simulink model "Microgrid_transition_model_111821_ben"  (R2020a)
settings: Solver=VariableStepAuto  StartTime=0.0  StopTime=20  MaxStep=1e-4  RelTol=1e-3
PreLoadFcn:
  | %run('FC_microgrid_param.m')
  | %load('gen_grid_init.mat')
InitFcn:
  | %load myisoModel_init;
  | run('FC_microgrid_param.m')
  | tic
  | run('CARTinitFcn.m')
  | %caseNo = 2;
  | 
  | %if (caseNo == 1)
  | %set_param(['Isolated_grid_paper_model_022521/SignalGen'], 'ActiveScenario', 'PStep222kW');
  | %else
  | %set_param(['Isolated_grid_paper_model_022521/SignalGen'], 'ActiveScenario', 'QStep222kVAr');
  | 
  | %end;
StopFcn:
  | toc
undefined symbols (not defined in the file): breakpoints1, breakpoints2, cc_kp, cp_table_data, ctrl, D1, Delta, DiscIntNeverNeededParam, DT, FC_BESS, FC_PV_FirstSolar, find_system, gcbh, libFC_BESS, libFC_PV, LowerLimit, magnitude, oversize, pll_ki, pll_kp, pq_ts, sps_rtmsupport, timer, ts, Ts, Ts_APC, Ts_Control, Ts_Power, UpperLimit
libraries: powerlib x152, powerlib_extras x100, simulink x95, powerlib_meascontrol x86, eePowerMeasurement x26, pi_ctrl x16, simulink_extras x12, sps_avr x7, spsDieselMotorModel x3, libFSArray x2, SignalEditorBlockLib x2, libLgBattery x1
(part 4 of 14)

== system Microgrid_transition_model_111821_ben/Defferable Load (0-446.25 kW)/Resistive Loads ==
  Bit 0 : powerlib/Elements/Three-Phase Parallel RLC Load  LConnTagsString=A|B|C  Configuration=Y (grounded)  NominalVoltage=Vphase_phase_lissage  Vabc=[1e3 1e3 1e3]  Vabcp=[1e3 1e3 1e3]  NominalFrequency=Freq  UnbalancedPower=off  ActivePower=P_lissage_min  InductivePower=0  CapacitivePower=0  Pabc=[10e3 9e3 11e3]  QLabc=[100 90 110]  QCabc=[100 90 110]  Pabcp=[10e3 9e3 11e3]  QLabcp=[100 90 110]  QCabcp=[100 90 110]  Measurements=None  LoadType=constant Z
      settings: SourceProductBaseCode=MT,PS
  Bit 1 : powerlib/Elements/Three-Phase Parallel RLC Load  LConnTagsString=A|B|C  Configuration=Y (grounded)  NominalVoltage=Vphase_phase_lissage  Vabc=[1e3 1e3 1e3]  Vabcp=[1e3 1e3 1e3]  NominalFrequency=Freq  UnbalancedPower=off  ActivePower=2*P_lissage_min  InductivePower=0  CapacitivePower=0  Pabc=[10e3 9e3 11e3]  QLabc=[100 90 110]  QCabc=[100 90 110]  Pabcp=[10e3 9e3 11e3]  QLabcp=[100 90 110]  QCabcp=[100 90 110]  Measurements=None  LoadType=constant Z
      settings: SourceProductBaseCode=MT,PS
  Bit 2 : powerlib/Elements/Three-Phase Parallel RLC Load  LConnTagsString=A|B|C  Configuration=Y (grounded)  NominalVoltage=Vphase_phase_lissage  Vabc=[1e3 1e3 1e3]  Vabcp=[1e3 1e3 1e3]  NominalFrequency=Freq  UnbalancedPower=off  ActivePower=2^2*P_lissage_min  InductivePower=0  CapacitivePower=0  Pabc=[10e3 9e3 11e3]  QLabc=[100 90 110]  QCabc=[100 90 110]  Pabcp=[10e3 9e3 11e3]  QLabcp=[100 90 110]  QCabcp=[100 90 110]  Measurements=None  LoadType=constant Z
      settings: SourceProductBaseCode=MT,PS
  Bit 3 : powerlib/Elements/Three-Phase Parallel RLC Load  LConnTagsString=A|B|C  Configuration=Y (grounded)  NominalVoltage=Vphase_phase_lissage  Vabc=[1e3 1e3 1e3]  Vabcp=[1e3 1e3 1e3]  NominalFrequency=Freq  UnbalancedPower=off  ActivePower=2^3*P_lissage_min  InductivePower=0  CapacitivePower=0  Pabc=[10e3 9e3 11e3]  QLabc=[100 90 110]  QCabc=[100 90 110]  Pabcp=[10e3 9e3 11e3]  QLabcp=[100 90 110]  QCabcp=[100 90 110]  Measurements=None  LoadType=constant Z
      settings: SourceProductBaseCode=MT,PS
  Bit 4 : powerlib/Elements/Three-Phase Parallel RLC Load  LConnTagsString=A|B|C  Configuration=Y (grounded)  NominalVoltage=Vphase_phase_lissage  Vabc=[1e3 1e3 1e3]  Vabcp=[1e3 1e3 1e3]  NominalFrequency=Freq  UnbalancedPower=off  ActivePower=2^4*P_lissage_min  InductivePower=0  CapacitivePower=0  Pabc=[10e3 9e3 11e3]  QLabc=[100 90 110]  QCabc=[100 90 110]  Pabcp=[10e3 9e3 11e3]  QLabcp=[100 90 110]  QCabcp=[100 90 110]  Measurements=None  LoadType=constant Z
      settings: SourceProductBaseCode=MT,PS
  Bit 5 : powerlib/Elements/Three-Phase Parallel RLC Load  LConnTagsString=A|B|C  Configuration=Y (grounded)  NominalVoltage=Vphase_phase_lissage  Vabc=[1e3 1e3 1e3]  Vabcp=[1e3 1e3 1e3]  NominalFrequency=Freq  UnbalancedPower=off  ActivePower=2^5*P_lissage_min  InductivePower=0  CapacitivePower=0  Pabc=[10e3 9e3 11e3]  QLabc=[100 90 110]  QCabc=[100 90 110]  Pabcp=[10e3 9e3 11e3]  QLabcp=[100 90 110]  QCabcp=[100 90 110]  Measurements=None  LoadType=constant Z
      settings: SourceProductBaseCode=MT,PS
  Bit 6 : powerlib/Elements/Three-Phase Parallel RLC Load  LConnTagsString=A|B|C  Configuration=Y (grounded)  NominalVoltage=Vphase_phase_lissage  Vabc=[1e3 1e3 1e3]  Vabcp=[1e3 1e3 1e3]  NominalFrequency=Freq  UnbalancedPower=off  ActivePower=2^6*P_lissage_min  InductivePower=0  CapacitivePower=0  Pabc=[10e3 9e3 11e3]  QLabc=[100 90 110]  QCabc=[100 90 110]  Pabcp=[10e3 9e3 11e3]  QLabcp=[100 90 110]  QCabcp=[100 90 110]  Measurements=None  LoadType=constant Z
      settings: SourceProductBaseCode=MT,PS
  Bit 7 : powerlib/Elements/Three-Phase Parallel RLC Load  LConnTagsString=A|B|C  Configuration=Y (grounded)  NominalVoltage=Vphase_phase_lissage  Vabc=[1e3 1e3 1e3]  Vabcp=[1e3 1e3 1e3]  NominalFrequency=Freq  UnbalancedPower=off  ActivePower=2^7*P_lissage_min  InductivePower=0  CapacitivePower=0  Pabc=[10e3 9e3 11e3]  QLabc=[100 90 110]  QCabc=[100 90 110]  Pabcp=[10e3 9e3 11e3]  QLabcp=[100 90 110]  QCabcp=[100 90 110]  Measurements=None  LoadType=constant Z
      settings: SourceProductBaseCode=MT,PS
  A0 : PMIOPort  Side=Left
  B0 : PMIOPort  Port=2  Side=Left
  C0 : PMIOPort  Port=3  Side=Left
  A1 : PMIOPort  Port=4  Side=Left
  B1 : PMIOPort  Port=5  Side=Left
  C1 : PMIOPort  Port=6  Side=Left
  A2 : PMIOPort  Port=7  Side=Left
  B2 : PMIOPort  Port=8  Side=Left
  C2 : PMIOPort  Port=9  Side=Left
  A3 : PMIOPort  Port=10  Side=Left
  B3 : PMIOPort  Port=11  Side=Left
  C3 : PMIOPort  Port=12  Side=Left
  A4 : PMIOPort  Port=13  Side=Left
  B4 : PMIOPort  Port=14  Side=Left
  C4 : PMIOPort  Port=15  Side=Left
  A5 : PMIOPort  Port=16  Side=Left
  B5 : PMIOPort  Port=17  Side=Left
  C5 : PMIOPort  Port=18  Side=Left
  A6 : PMIOPort  Port=19  Side=Left
  B6 : PMIOPort  Port=20  Side=Left
  C6 : PMIOPort  Port=21  Side=Left
  A7 : PMIOPort  Port=22  Side=Left
  B7 : PMIOPort  Port=23  Side=Left
  C7 : PMIOPort  Port=24  Side=Left
  connections:
  C7/RConn1 -- Bit 7/LConn3
  B7/RConn1 -- Bit 7/LConn2
  A7/RConn1 -- Bit 7/LConn1
  C6/RConn1 -- Bit 6/LConn3
  B6/RConn1 -- Bit 6/LConn2
  A6/RConn1 -- Bit 6/LConn1
  C5/RConn1 -- Bit 5/LConn3
  B5/RConn1 -- Bit 5/LConn2
  A5/RConn1 -- Bit 5/LConn1
  C4/RConn1 -- Bit 4/LConn3
  B4/RConn1 -- Bit 4/LConn2
  A4/RConn1 -- Bit 4/LConn1
  C3/RConn1 -- Bit 3/LConn3
  B3/RConn1 -- Bit 3/LConn2
  A3/RConn1 -- Bit 3/LConn1
  C2/RConn1 -- Bit 2/LConn3
  B2/RConn1 -- Bit 2/LConn2
  A2/RConn1 -- Bit 2/LConn1
  C1/RConn1 -- Bit 1/LConn3
  B1/RConn1 -- Bit 1/LConn2
  A1/RConn1 -- Bit 1/LConn1
  C0/RConn1 -- Bit 0/LConn3
  B0/RConn1 -- Bit 0/LConn2
  A0/RConn1 -- Bit 0/LConn1

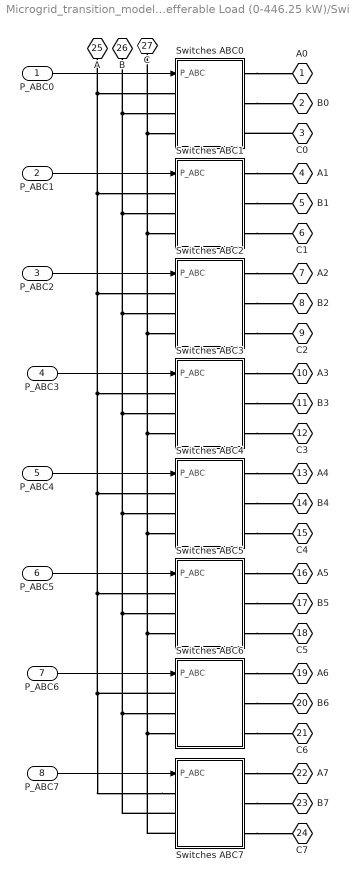
== system Microgrid_transition_model_111821_ben/Defferable Load (0-446.25 kW)/Switches ==
  P_ABC0 : Inport
  P_ABC1 : Inport  Port=2
  P_ABC2 : Inport  Port=3
  P_ABC3 : Inport  Port=4
  P_ABC4 : Inport  Port=5
  P_ABC5 : Inport  Port=6
  P_ABC6 : Inport  Port=7
  P_ABC7 : Inport  Port=8
  Switches ABC0 : Subsystem
  Switches ABC1 : Subsystem
  Switches ABC2 : Subsystem
  Switches ABC3 : Subsystem
  Switches ABC4 : Subsystem
  Switches ABC5 : Subsystem
  Switches ABC6 : Subsystem
  Switches ABC7 : Subsystem
  A0 : PMIOPort  Side=Right
  B0 : PMIOPort  Port=2  Side=Right
  C0 : PMIOPort  Port=3  Side=Right
  A1 : PMIOPort  Port=4  Side=Right
  B1 : PMIOPort  Port=5  Side=Right
  C1 : PMIOPort  Port=6  Side=Right
  A2 : PMIOPort  Port=7  Side=Right
  B2 : PMIOPort  Port=8  Side=Right
  C2 : PMIOPort  Port=9  Side=Right
  A3 : PMIOPort  Port=10  Side=Right
  B3 : PMIOPort  Port=11  Side=Right
  C3 : PMIOPort  Port=12  Side=Right
  A4 : PMIOPort  Port=13  Side=Right
  B4 : PMIOPort  Port=14  Side=Right
  C4 : PMIOPort  Port=15  Side=Right
  A5 : PMIOPort  Port=16  Side=Right
  B5 : PMIOPort  Port=17  Side=Right
  C5 : PMIOPort  Port=18  Side=Right
  A6 : PMIOPort  Port=19  Side=Right
  B6 : PMIOPort  Port=20  Side=Right
  C6 : PMIOPort  Port=21  Side=Right
  A7 : PMIOPort  Port=22  Side=Right
  B7 : PMIOPort  Port=23  Side=Right
  C7 : PMIOPort  Port=24  Side=Right
  A : PMIOPort  Port=25  Side=Left
  B : PMIOPort  Port=26  Side=Left
  C : PMIOPort  Port=27  Side=Left
  wires:
  P_ABC7/1 -> Switches ABC7/1(P_ABC)
  P_ABC6/1 -> Switches ABC6/1(P_ABC)
  P_ABC5/1 -> Switches ABC5/1(P_ABC)
  P_ABC4/1 -> Switches ABC4/1(P_ABC)
  P_ABC3/1 -> Switches ABC3/1(P_ABC)
  P_ABC2/1 -> Switches ABC2/1(P_ABC)
  P_ABC1/1 -> Switches ABC1/1(P_ABC)
  P_ABC0/1 -> Switches ABC0/1(P_ABC)
  connections:
  Switches ABC0/RConn1 -- A0/RConn1
  Switches ABC0/RConn2 -- B0/RConn1
  C0/RConn1 -- Switches ABC0/RConn3
  Switches ABC1/RConn1 -- A1/RConn1
  Switches ABC1/RConn2 -- B1/RConn1
  Switches ABC1/RConn3 -- C1/RConn1
  Switches ABC2/RConn1 -- A2/RConn1
  Switches ABC2/RConn2 -- B2/RConn1
  Switches ABC2/RConn3 -- C2/RConn1
  Switches ABC3/RConn1 -- A3/RConn1
  Switches ABC3/RConn2 -- B3/RConn1
  Switches ABC3/RConn3 -- C3/RConn1
  Switches ABC4/RConn1 -- A4/RConn1
  Switches ABC4/RConn2 -- B4/RConn1
  Switches ABC4/RConn3 -- C4/RConn1
  Switches ABC5/RConn1 -- A5/RConn1
  Switches ABC5/RConn2 -- B5/RConn1
  Switches ABC5/RConn3 -- C5/RConn1
  Switches ABC6/RConn1 -- A6/RConn1
  Switches ABC6/RConn2 -- B6/RConn1
  Switches ABC6/RConn3 -- C6/RConn1
  Switches ABC7/RConn3 -- C7/RConn1
  Switches ABC7/RConn2 -- B7/RConn1
  Switches ABC7/RConn1 -- A7/RConn1
  Switches ABC7/LConn2 -- Switches ABC0/LConn2 -- B/RConn1 -- Switches ABC1/LConn2 -- Switches ABC2/LConn2 -- Switches ABC3/LConn2 -- Switches ABC4/LConn2 -- Switches ABC5/LConn2 -- Switches ABC6/LConn2
  Switches ABC7/LConn3 -- Switches ABC0/LConn3 -- C/RConn1 -- Switches ABC1/LConn3 -- Switches ABC2/LConn3 -- Switches ABC3/LConn3 -- Switches ABC4/LConn3 -- Switches ABC5/LConn3 -- Switches ABC6/LConn3
  Switches ABC7/LConn1 -- Switches ABC0/LConn1 -- A/RConn1 -- Switches ABC1/LConn1 -- Switches ABC2/LConn1 -- Switches ABC3/LConn1 -- Switches ABC4/LConn1 -- Switches ABC5/LConn1 -- Switches ABC6/LConn1

== system Microgrid_transition_model_111821_ben/Discrete Frequency Regulator/Discrete PID Controller ==
  note: Pierre Giroux, Gilbert Sybille
      | Power System Simulation Laboratory
      | IREQ, Hydro-Quebc
  note: Discrete PID Controller
  Error : Inport  SampleTime=Ts
  "Derivative " : DiscreteTransferFcn  Numerator=[2 -2]  Denominator=[Ts+2*TcD Ts-2*TcD]  SampleTime=Ts
  Discrete-Time Integrator : DiscreteIntegrator  InitialCondition=Init  SampleTime=Ts  LimitOutput=on  UpperSaturationLimit=UpperLimit  LowerSaturationLimit=LowerLimit  ICPrevOutput=DiscIntNeverNeededParam  ICPrevScaledInput=DiscIntNeverNeededParam
  Kp4 : Gain  Gain=Kp  SaturateOnIntegerOverflow=on  SampleTime=Ts  OutDataTypeStr=Inherit: Same as input  ParamDataTypeStr=Inherit: Same as input
  Kp5 : Gain  Gain=Ki  SaturateOnIntegerOverflow=on  SampleTime=Ts  OutDataTypeStr=Inherit: Same as input  ParamDataTypeStr=Inherit: Same as input
  Kp6 : Gain  Gain=Kd  SaturateOnIntegerOverflow=on  SampleTime=Ts  OutDataTypeStr=Inherit: Same as input  ParamDataTypeStr=Inherit: Same as input
  Saturation2 : Saturate  UpperLimit=UpperLimit  LowerLimit=LowerLimit  SampleTime=Ts
  Sum6 : Sum  Inputs=+++  InputSameDT=on  SaturateOnIntegerOverflow=on  SampleTime=Ts  OutDataTypeStr=Inherit: Same as first input
  Zero-Order Hold : ZeroOrderHold  SampleTime=Ts
  Out : Outport  SampleTime=Ts  InitialOutput=0  VectorParamsAs1DForOutWhenUnconnected=off
  wires:
  Saturation2/1 -> Out/1
  Error/1 -> Kp4/1, Kp5/1, Kp6/1
  Sum6/1 -> Saturation2/1
  Kp5/1 -> Discrete-Time Integrator/1
  Kp6/1 -> "Derivative "/1
  Kp4/1 -> Zero-Order Hold/1
  Discrete-Time Integrator/1 -> Sum6/2
  "Derivative "/1 -> Sum6/3
  Zero-Order Hold/1 -> Sum6/1

== system Microgrid_transition_model_111821_ben/Discrete Frequency Regulator/Pulses Decoder ==
  Code : Inport
  Constant : Constant  Value=pow2(0:-1:-(n-1))
  Constant6 : Constant  Value=2
  Math Function : Math  Operator=rem  SignedPower=on  SaturateOnIntegerOverflow=on
  Product : Product  InputSameDT=on  SaturateOnIntegerOverflow=on  OutDataTypeStr=Inherit: Same as first input
  Rounding Function : Rounding
  Pulses : Outport  VectorParamsAs1DForOutWhenUnconnected=off
  wires:
  Math Function/1 -> Pulses/1
  Rounding Function/1 -> Math Function/1
  Constant6/1 -> Math Function/2
  Product/1 -> Rounding Function/1
  Code/1 -> Product/1
  Constant/1 -> Product/2

== system Microgrid_transition_model_111821_ben/Discrete Frequency Regulator/Sampling system ==
  note: T_ABC7
  note: T_ABC6
  note: T_ABC5
  note: T_ABC4
  note: T_ABC3
  note: T_ABC2
  note: T_ABC1
  note: T_ABC0
  note: Tc0_7
  note: Tb0_7
  note: Ta0_7
  BITA0_7 : Inport
  " Bit ABC4" : Selector  InputPortWidth=24  IndexOptions=Index vector (dialog)  Indices=[13 14 15]  OutputSizes=1
  Bit ABC0 : Selector  InputPortWidth=24  IndexOptions=Index vector (dialog)  Indices=[1 2 3]  OutputSizes=1
  Bit ABC1 : Selector  InputPortWidth=24  IndexOptions=Index vector (dialog)  Indices=[4 5 6]  OutputSizes=1
  Bit ABC2 : Selector  InputPortWidth=24  IndexOptions=Index vector (dialog)  Indices=[7 8 9]  OutputSizes=1
  Bit ABC3 : Selector  InputPortWidth=24  IndexOptions=Index vector (dialog)  Indices=[10 11 12]  OutputSizes=1
  Bit ABC5 : Selector  InputPortWidth=24  IndexOptions=Index vector (dialog)  Indices=[16 17 18]  OutputSizes=1
  Bit ABC6 : Selector  InputPortWidth=24  IndexOptions=Index vector (dialog)  Indices=[19 20 21]  OutputSizes=1
  Bit ABC7 : Selector  InputPortWidth=24  IndexOptions=Index vector (dialog)  Indices=[22 23 24]  OutputSizes=1
  Demux : Demux  Outputs=3
      settings: DisplayOption=none
  Mux : Mux  Inputs=3
  Mux1 : Mux  Inputs=8
  Selector : Selector  InputPortWidth=24  IndexOptions=Index vector (dialog)  Indices=[1 9 17 2 10 18 3 11 19 4 12 20 5 13 21 6 14 22 7 15 23 8 16 24]  OutputSizes=1
  Switch : Switch  Threshold=0.5  SaturateOnIntegerOverflow=on  InputSameDT=on
  Switch1 : Switch  Threshold=0.5  SaturateOnIntegerOverflow=on  InputSameDT=on
  Switch2 : Switch  Threshold=0.5  SaturateOnIntegerOverflow=on  InputSameDT=on
  Unit Delay{,1..2,4..6} (6 alike) : UnitDelay  SampleTime=Ts  HasFrameUpgradeWarning=on
  Zero crossing : HitCross
  Zero crossing1 : HitCross
  Zero crossing2 : HitCross
  Pulses_ABC0_7 : Outport  VectorParamsAs1DForOutWhenUnconnected=off
  wires:
  BITA0_7/1 -> Switch2/1, Switch1/1, Switch/1
  Demux/3 -> Unit Delay2/1
  Demux/2 -> Unit Delay1/1
  Demux/1 -> Unit Delay/1
  Mux1/1 -> Pulses_ABC0_7/1
  Bit ABC7/1 -> Mux1/8
  Bit ABC6/1 -> Mux1/7
  Bit ABC5/1 -> Mux1/6
  " Bit ABC4"/1 -> Mux1/5
  Bit ABC3/1 -> Mux1/4
  Bit ABC2/1 -> Mux1/3
  Bit ABC1/1 -> Mux1/2
  Bit ABC0/1 -> Mux1/1
  Selector/1 -> Bit ABC7/1, Bit ABC6/1, Bit ABC5/1, " Bit ABC4"/1, Bit ABC3/1, Bit ABC2/1, Bit ABC0/1, Bit ABC1/1
  Mux/1 -> Selector/1
  Unit Delay6/1 -> Switch2/3
  Switch2/1 -> Mux/3, Unit Delay6/1
  Unit Delay5/1 -> Switch1/3
  Switch1/1 -> Mux/2, Unit Delay5/1
  Unit Delay4/1 -> Switch/3
  Switch/1 -> Mux/1, Unit Delay4/1
  Unit Delay/1 -> Zero crossing/1
  Unit Delay2/1 -> Zero crossing2/1
  Zero crossing/1 -> Switch/2
  Zero crossing1/1 -> Switch1/2
  Zero crossing2/1 -> Switch2/2
  [Vabc_SL] -> Demux/1
  Unit Delay1/1 -> Zero crossing1/1

== system Microgrid_transition_model_111821_ben/FC_BESS/Battery ==
  Idc : Inport
  LG_Battery : libLgBattery/LG_Battery  SystemSampleTime=-1  Latency=0  AutoFrameSizeCalculation=off
  Vdc : Outport
  m : Outport  Port=2
  wires:
  Idc/1 -> LG_Battery/1
  LG_Battery/1 -> Vdc/1
  LG_Battery/2 -> m/1

== system Microgrid_transition_model_111821_ben/FC_BESS/SMAInverter ==
  Vdc : Inport
  Control : Inport  Port=2
  85_SMAControl : Subsystem
  Add : Sum  Inputs=--
  BESS Inverter : Subsystem
  Bus Selector2 : BusSelector  OutputSignals=ToCB,Uabc
  Bus Selector4 : BusSelector  OutputSignals=Close
  Divide : Product  Inputs=*/
  Goto Tag Visibility : GotoTagVisibility  GotoTag=Ugri
  Goto Tag Visibility1 : GotoTagVisibility  GotoTag=Igri
  Goto Tag Visibility4 : GotoTagVisibility  GotoTag=Iinv
  Goto Tag Visibility5 : GotoTagVisibility  GotoTag=Uinv
  Inverter Filter : powerlib/Elements/Three-Phase Parallel RLC Load  LConnTagsString=A|B|C  Configuration=Y (grounded)  NominalVoltage=400  Vabc=[1e3 1e3 1e3]  Vabcp=[1e3 1e3 1e3]  NominalFrequency=60  UnbalancedPower=off  ActivePower=4e3  InductivePower=0  CapacitivePower=233^2/(1/2/pi/60/444e-6/3)  Pabc=[10e3 9e3 11e3]  QLabc=[100 90 110]  QCabc=[100 90 110]  Pabcp=[10e3 9e3 11e3]  QLabcp=[100 90 110]  QCabcp=[100 90 110]  Measurements=Branch voltages and currents  LoadType=constant Z
  InverterLosses : Constant  Value=5000
  Neutral1 : powerlib/Elements/Neutral  LConnTagsString=a  NodeNumber=10
      settings: SourceProductBaseCode=PS
  "Power (3ph, Instantaneous)" : powerlib_meascontrol/Measurements/Power (3ph, Instantaneous)
  Power Measurement (Three-Phase) : eePowerMeasurement/Power Measurement (Three-Phase)  LabelModeActiveChoice=Continuous  F=60  K=[1]  Seq=Positive  Ts=0
      settings: SourceProductBaseCode=PS
  Saturation : Saturate  UpperLimit=2000  LowerLimit=500
  Scope : Scope  Commented=on  NumInputPorts=3
  Scope1 : Scope  Commented=on  NumInputPorts=4
  Sine Filter : powerlib/Elements/Three-Phase Series RLC Branch  LConnTagsString=A|B|C  RConnTagsString=A|B|C  BranchType=RL  Resistance=0.003  Inductance=48e-6  Capacitance=1e-6  Measurements=None
  SmaBreaker : powerlib/Elements/Three-Phase Breaker  InitialState=open  SwitchA=on  SwitchB=on  SwitchC=on  SwitchTimes="[4/60  10/60]"  External=on  BreakerResistance=0.000001  SnubberResistance=1e6  SnubberCapacitance=inf  Measurements=None
  Subsystem : Subsystem
  Subsystem1 : Subsystem
  Terminator : Terminator
  Terminator2 : Terminator
  a : PMIOPort  Side=Left
  b : PMIOPort  Port=2  Side=Left
  c : PMIOPort  Port=3  Side=Left
  Idc : Outport
  wires:
  Vdc/1 -> Saturation/1
  InverterLosses/1 -> Add/2
  [Ugri] -> "Power (3ph, Instantaneous)"/1
  [Igri] -> "Power (3ph, Instantaneous)"/2
  Add/1 -> Divide/1  "Pdc"
  Divide/1 -> Idc/1  "Idc"
  "Power (3ph, Instantaneous)"/2 -> Terminator/1
  "Power (3ph, Instantaneous)"/1 -> Add/1
  Saturation/1 -> Divide/2
  [Igri] -> Scope/3
  [circuit_Usmainv] -> Scope/2
  [Ugri] -> Scope/1
  [Igri] -> 85_SMAControl/3(Iabc)
  [Ugri] -> 85_SMAControl/1(Uabc)
  Bus Selector2/1 -> Bus Selector4/1  "<ToCB>"
  Bus Selector4/1 -> SmaBreaker/1, 85_SMAControl/4(CB_status)  "<Close>"
  Bus Selector2/2 -> BESS Inverter/1(ctrl)  "<Uabc>"
  85_SMAControl/1(CtrlOut) -> Bus Selector2/1
  [Iinv] -> Terminator2/1
  Control/1 -> 85_SMAControl/5(Control)
  [Uinv] -> 85_SMAControl/2(Uabc_inv)
  [Iinv] -> Scope1/3, Power Measurement (Three-Phase)/1
  [Uinv] -> Scope1/4, Power Measurement (Three-Phase)/2
  Power Measurement (Three-Phase)/1 -> Scope1/1
  Power Measurement (Three-Phase)/2 -> Scope1/2
  connections:
  Neutral1/LConn1 -- BESS Inverter/LConn1
  Sine Filter/LConn3 -- BESS Inverter/RConn3
  Sine Filter/LConn1 -- BESS Inverter/RConn1
  BESS Inverter/RConn2 -- Sine Filter/LConn2
  Subsystem/LConn1 -- SmaBreaker/RConn1
  Subsystem/LConn2 -- SmaBreaker/RConn2
  Subsystem/RConn1 -- a/RConn1
  Subsystem/RConn2 -- b/RConn1
  Subsystem/LConn3 -- SmaBreaker/RConn3
  Subsystem/RConn3 -- c/RConn1
  Subsystem1/LConn2 -- Sine Filter/RConn2 -- Inverter Filter/LConn2
  Sine Filter/RConn1 -- Subsystem1/LConn1 -- Inverter Filter/LConn1
  Sine Filter/RConn3 -- Subsystem1/LConn3 -- Inverter Filter/LConn3
  Subsystem1/RConn1 -- SmaBreaker/LConn1
  Subsystem1/RConn2 -- SmaBreaker/LConn2
  Subsystem1/RConn3 -- SmaBreaker/LConn3

== system Microgrid_transition_model_111821_ben/FC_PV_FirstSolar/AllStringInverters ==
  Idc : Inport
  Control : Inport  Port=2
  BESS Inverter : Subsystem
  Bus Selector2 : BusSelector  OutputSignals=ToCB,Uabc
  Bus Selector4 : BusSelector  OutputSignals=Close
  Constant : Constant  Value=1000
  Divide : Product  Inputs=**
  Gain : Gain  Gain=1/430e3
  Goto Tag Visibility : GotoTagVisibility  GotoTag=Ugri
  Goto Tag Visibility1 : GotoTagVisibility  GotoTag=Igri
  Goto Tag Visibility4 : GotoTagVisibility  GotoTag=Iinv
  Goto Tag Visibility5 : GotoTagVisibility  GotoTag=Uinv
  Inverter Filter : powerlib/Elements/Three-Phase Parallel RLC Load  LConnTagsString=A|B|C  Configuration=Y (grounded)  NominalVoltage=400  Vabc=[1e3 1e3 1e3]  Vabcp=[1e3 1e3 1e3]  NominalFrequency=60  UnbalancedPower=off  ActivePower=1e3  InductivePower=0  CapacitivePower=0.2*346^2/(1/2/pi/60/444e-6/3)  Pabc=[10e3 9e3 11e3]  QLabc=[100 90 110]  QCabc=[100 90 110]  Pabcp=[10e3 9e3 11e3]  QLabcp=[100 90 110]  QCabcp=[100 90 110]  Measurements=Branch voltages and currents  LoadType=constant Z
  Neutral1 : powerlib/Elements/Neutral  LConnTagsString=a  NodeNumber=10
      settings: SourceProductBaseCode=PS
  PV_Control : Subsystem
  Power Measurement (Three-Phase)1 : eePowerMeasurement/Power Measurement (Three-Phase)  LabelModeActiveChoice=Discrete  F=60  K=[1]  Seq=Positive  Ts=Ts
      settings: SourceProductBaseCode=PS
  Power Measurement (Three-Phase)2 : eePowerMeasurement/Power Measurement (Three-Phase)  LabelModeActiveChoice=Discrete  F=60  K=[1]  Seq=Positive  Ts=Ts
      settings: SourceProductBaseCode=PS
  Scope : Scope  NumInputPorts=3
  Scope2 : Scope  NumInputPorts=2
  Scope4 : Scope  NumInputPorts=2
  Scope5 : Scope
  Sine Filter : powerlib/Elements/Three-Phase Series RLC Branch  LConnTagsString=A|B|C  RConnTagsString=A|B|C  BranchType=RL  Resistance=0.003*2  Inductance=48e-6*2  Capacitance=1e-6  Measurements=None
  SmaBreaker : powerlib/Elements/Three-Phase Breaker  InitialState=open  SwitchA=on  SwitchB=on  SwitchC=on  SwitchTimes="[4/60  10/60]"  External=on  BreakerResistance=0.000001  SnubberResistance=1e6  SnubberCapacitance=inf  Measurements=None
  Subsystem1 : Subsystem
  Subsystem2 : Subsystem
  Terminator3 : Terminator
  a : PMIOPort  Side=Left
  b : PMIOPort  Port=2  Side=Left
  c : PMIOPort  Port=3  Side=Left
  Udc : Outport
  wires:
  [Uinv] -> PV_Control/2(Uabc_inv)
  Control/1 -> PV_Control/5(Control)
  PV_Control/1(CtrlOut) -> Bus Selector2/1
  Bus Selector2/2 -> BESS Inverter/1(ctrl)  "<Uabc>"
  Bus Selector4/1 -> PV_Control/4(CB_status), SmaBreaker/1  "<Close>"
  Bus Selector2/1 -> Bus Selector4/1  "<ToCB>"
  [Ugri] -> PV_Control/1(Uabc)
  [Igri] -> PV_Control/3(Iabc)
  [Ugri] -> Scope/1
  [Uinv] -> Scope/2
  [Igri] -> Scope/3
  Idc/1 -> Divide/2
  Divide/1 -> Gain/1  "Ppv"
  Constant/1 -> Divide/1, Udc/1  "Udc"
  [Iinv] -> Terminator3/1
  Gain/1 -> Scope5/1, PV_Control/6(Ppv)
  [Ugri] -> Power Measurement (Three-Phase)1/1
  Power Measurement (Three-Phase)1/1 -> Scope2/1  "Psolar"
  Power Measurement (Three-Phase)1/2 -> Scope2/2  "Q4"
  [Igri] -> Power Measurement (Three-Phase)1/2
  Power Measurement (Three-Phase)2/1 -> Scope4/1  "Psolar"
  Power Measurement (Three-Phase)2/2 -> Scope4/2  "Q4"
  [Uinv] -> Power Measurement (Three-Phase)2/1
  [Iinv] -> Power Measurement (Three-Phase)2/2
  connections:
  Subsystem1/RConn2 -- SmaBreaker/LConn2
  BESS Inverter/RConn2 -- Sine Filter/LConn2
  Subsystem1/LConn2 -- Sine Filter/RConn2 -- Inverter Filter/LConn2
  Sine Filter/LConn1 -- BESS Inverter/RConn1
  Subsystem2/LConn3 -- SmaBreaker/RConn3
  Subsystem2/LConn1 -- SmaBreaker/RConn1
  Subsystem2/RConn3 -- c/RConn1
  Sine Filter/LConn3 -- BESS Inverter/RConn3
  Subsystem1/RConn3 -- SmaBreaker/LConn3
  Subsystem1/RConn1 -- SmaBreaker/LConn1
  Sine Filter/RConn3 -- Subsystem1/LConn3 -- Inverter Filter/LConn3
  Neutral1/LConn1 -- BESS Inverter/LConn1
  Subsystem2/LConn2 -- SmaBreaker/RConn2
  Sine Filter/RConn1 -- Subsystem1/LConn1 -- Inverter Filter/LConn1
  Subsystem2/RConn1 -- a/RConn1
  Subsystem2/RConn2 -- b/RConn1

== system Microgrid_transition_model_111821_ben/FC_PV_FirstSolar/MPPT Parameters ==
  note: Parameters for Perturb and Observe Algorithm:
  note: Lower limit for Vdc_ref (Dmax)
  note: Initial value for Vdc_ref output (Dinit)
  note: Increment value used to increase/decrease Vdc_ref (DeltaD)
  note: Upper limit for Vdc_ref (Dmax)
  Iph_ : Constant  Value=Vdc_ref_Init
  Iph_1 : Constant  Value=Limits_MPPT(1)
  Iph_2 : Constant  Value=Limits_MPPT(2)
  Iph_3 : Constant  Value=Increment_MPPT
  Mux : Mux
  Param : Outport  VectorParamsAs1DForOutWhenUnconnected=off
  wires:
  Mux/1 -> Param/1
  Iph_3/1 -> Mux/4
  Iph_2/1 -> Mux/3
  Iph_1/1 -> Mux/2
  Iph_/1 -> Mux/1

== system Microgrid_transition_model_111821_ben/FC_PV_FirstSolar/PV_Array ==
  Vdc : Inport
  Irradiance : Inport  Port=2
  FS_Array : libFSArray/FS_Array  SystemSampleTime=-1  Latency=0  AutoFrameSizeCalculation=off
  Idc : Outport
  m : Outport  Port=2
  wires:
  Vdc/1 -> FS_Array/1
  Irradiance/1 -> FS_Array/2
  FS_Array/1 -> Idc/1
  FS_Array/2 -> m/1

== system Microgrid_transition_model_111821_ben/Grid Feeder Protective Relay/CS Modified PLL ==
  note: Pierre Giroux, Gilbert Sybille
      | Power System Laboratory, IREQ
      | Hydro-Quebec
      | (August 2007)
  note: SPS Discrete 3-phase PLL
  Vabc(pu) : Inport  PortDimensions=3
  2nd-Order Filter : powerlib_extras/Discrete  Control Blocks/Discrete  2nd-Order Filter  FilterType=Lowpass  Fo=25  Zeta=0.707  Ts=Ts  Initialize=on  Vac_Init=[0 0 Finit]  Vdc_Init=Finit  PlotResponse=off  param1=[1 500 0.1]
      settings: SourceProductBaseCode=PS
  Controller : Subsystem  mask(Discrete PID Controller){Kp=Kp, Ki=Ki, Kd=Kd, Par_Limits=[Flim(2) Flim(1)]*2*pi, Init=2*pi*Finit, Ts=Ts}
      mask prompts: Kp "Proportional gain (Kp):"; Ki "Integral gain (Ki):"; Kd "Derivative gain (Kd):"; Par_Limits "Output limits: [ Upper   Lower ]"; Init "Output initial value:"; Ts "Sample time:"
      mask help: This block implements a discrete PID controller.
      mask init:
      | UpperLimit=Par_Limits(1);
      | LowerLimit=Par_Limits(2);
      | power_initmask();
      settings: OpenFcn=power_openblockproxy();
      mask Display: disp('PID');
  Discrete Rate Limiter : powerlib_extras/Discrete  Control Blocks/Discrete Rate Limiter  R=12  F=-12  Vinit=Finit  Ts=Ts
      settings: SourceProductBaseCode=PS
  Discrete Mean value : powerlib_extras/Discrete Measurements/Discrete  Mean value  Freq=60  Vinit=0  Ts=Ts
      settings: SourceProductBaseCode=PS
  Gain10 : Gain  Gain=1/2/pi  SaturateOnIntegerOverflow=on  OutDataTypeStr=Inherit: Same as input  ParamDataTypeStr=Inherit: Same as input
  Mux2 : Mux  Inputs=2
  Selector : Selector  InputPortWidth=3  IndexOptions=Index vector (dialog)  Indices=2  OutputSizes=1
  Trigonometric Function : Trigonometry
  Trigonometric Function2 : Trigonometry  Operator=cos
  Unit Delay : UnitDelay  InitialCondition=Finit  SampleTime=Ts  HasFrameUpgradeWarning=on
  VCO : Subsystem
  abc_to_dq0 Transformation : powerlib_extras/Measurements/abc_to_dq0 Transformation
      settings: SourceProductBaseCode=PS
  Freq : Outport
  wt : Outport  Port=2
  Sin_Cos : Outport  Port=3
  wires:
  Selector/1 -> Discrete Mean value/1  "Vq"
  2nd-Order Filter/1 -> Unit Delay/1
  Unit Delay/1 -> Freq/1
  Discrete Rate Limiter/1 -> 2nd-Order Filter/1
  Gain10/1 -> Discrete Rate Limiter/1
  Mux2/1 -> Sin_Cos/1, abc_to_dq0 Transformation/2
  Trigonometric Function2/1 -> Mux2/2
  Trigonometric Function/1 -> Mux2/1
  VCO/1(theta) -> wt/1, Trigonometric Function2/1, Trigonometric Function/1
  abc_to_dq0 Transformation/1 -> Selector/1
  Vabc(pu)/1 -> abc_to_dq0 Transformation/1
  Controller/1(Out) -> Gain10/1, VCO/1(w)  "W"
  Discrete Mean value/1 -> Controller/1(Error)

== system Microgrid_transition_model_111821_ben/Grid Feeder Protective Relay/CS Modified PLL1 ==
  note: Pierre Giroux, Gilbert Sybille
      | Power System Laboratory, IREQ
      | Hydro-Quebec
      | (August 2007)
  note: SPS Discrete 3-phase PLL
  Vabc(pu) : Inport  PortDimensions=3
  2nd-Order Filter : powerlib_extras/Discrete  Control Blocks/Discrete  2nd-Order Filter  FilterType=Lowpass  Fo=25  Zeta=0.707  Ts=Ts  Initialize=on  Vac_Init=[0 0 Finit]  Vdc_Init=Finit  PlotResponse=off  param1=[1 500 0.1]
      settings: SourceProductBaseCode=PS
  Controller : Subsystem  mask(Discrete PID Controller){Kp=Kp, Ki=Ki, Kd=Kd, Par_Limits=[Flim(2) Flim(1)]*2*pi, Init=2*pi*Finit, Ts=Ts}
      mask prompts: Kp "Proportional gain (Kp):"; Ki "Integral gain (Ki):"; Kd "Derivative gain (Kd):"; Par_Limits "Output limits: [ Upper   Lower ]"; Init "Output initial value:"; Ts "Sample time:"
      mask help: This block implements a discrete PID controller.
      mask init:
      | UpperLimit=Par_Limits(1);
      | LowerLimit=Par_Limits(2);
      | power_initmask();
      settings: OpenFcn=power_openblockproxy();
      mask Display: disp('PID');
  Discrete Rate Limiter : powerlib_extras/Discrete  Control Blocks/Discrete Rate Limiter  R=12  F=-12  Vinit=Finit  Ts=Ts
      settings: SourceProductBaseCode=PS
  Discrete Mean value : powerlib_extras/Discrete Measurements/Discrete  Mean value  Freq=60  Vinit=0  Ts=Ts
      settings: SourceProductBaseCode=PS
  Gain10 : Gain  Gain=1/2/pi  SaturateOnIntegerOverflow=on  OutDataTypeStr=Inherit: Same as input  ParamDataTypeStr=Inherit: Same as input
  Mux2 : Mux  Inputs=2
  Selector : Selector  InputPortWidth=3  IndexOptions=Index vector (dialog)  Indices=2  OutputSizes=1
  Trigonometric Function : Trigonometry
  Trigonometric Function2 : Trigonometry  Operator=cos
  Unit Delay : UnitDelay  InitialCondition=Finit  SampleTime=Ts  HasFrameUpgradeWarning=on
  VCO : Subsystem
  abc_to_dq0 Transformation : powerlib_extras/Measurements/abc_to_dq0 Transformation
      settings: SourceProductBaseCode=PS
  Freq : Outport
  wt : Outport  Port=2
  Sin_Cos : Outport  Port=3
  wires:
  Selector/1 -> Discrete Mean value/1  "Vq"
  2nd-Order Filter/1 -> Unit Delay/1
  Unit Delay/1 -> Freq/1
  Discrete Rate Limiter/1 -> 2nd-Order Filter/1
  Gain10/1 -> Discrete Rate Limiter/1
  Mux2/1 -> Sin_Cos/1, abc_to_dq0 Transformation/2
  Trigonometric Function2/1 -> Mux2/2
  Trigonometric Function/1 -> Mux2/1
  VCO/1(theta) -> wt/1, Trigonometric Function2/1, Trigonometric Function/1
  abc_to_dq0 Transformation/1 -> Selector/1
  Vabc(pu)/1 -> abc_to_dq0 Transformation/1
  Controller/1(Out) -> Gain10/1, VCO/1(w)  "W"
  Discrete Mean value/1 -> Controller/1(Error)

== system Microgrid_transition_model_111821_ben/Grid Feeder Protective Relay/R25 - Sync Check v0.1 ==
  note: * this block checks for synchronism based on phase A only
      | * the block also implements a deadbus logic
  note: angle difference
  note: frequency difference
  note: voltage difference
  note: true: If the life bus has voltage > 0.9pu and the other bus has voltage < threshold
      | true: both sides of the breaker are deadbuses
  note: Copyright 2018 Alliance for Sustainable Energy, LLC
      |
      | Permission is hereby granted, free of charge, to any person obtaining a copy of this software
      | and associated documentation files (the "Software"), to deal in the Software without restriction,
      | including without limitation the rights to use, copy, modify, merge, publish, distribute, sublicense,
      | and/or sell copies of the Software, and to permit persons to whom the Software is furnished to do so,
      | subject to the following conditions:
      |
      | The above copyright notice and this permission notice shall be included in all copies or substantial portions of the Software.
      |
      | THE SOFTWARE IS PROVIDED "AS IS", WITHOUT WARRANTY OF ANY KIND, EXPRESS OR IMPLIED, INCLUDING
      | BUT NOT LIMITED TO THE WARRANTIES OF MERCHANTABILITY, FITNESS FOR A PARTICULAR PURPOSE AND
      | NONINFRINGEMENT. IN NO EVENT SHALL THE AUTHORS, THE COPYRIGHT HOLDERS, THE UNITED STATES,
      | THE UNITED STATES DEPARTMENT OF ENERGY, OR ANY OF THEIR EMPLOYEES BE LIABLE FOR ANY CLAIM,
      | DAMAGES OR OTHER LIABILITY, WHETHER IN AN ACTION OF CONTRACT, TORT OR OTHERWISE, ARISING FROM,
      | OUT OF OR IN CONNECTION WITH THE SOFTWARE OR THE USE OR OTHER DEALINGS IN THE SOFTWARE.
  VPKLN_bus : Inport
  VPKLN_line : Inport  Port=2
  pll_data : Inport  Port=3
  relay_param : Inport  Port=4
  Bus Creator : BusCreator  Inputs=3
  Bus Selector : BusSelector  OutputSignals=VRMSLL,dV_threshold,angle_threshold,dF_threshold
  Bus Selector1 : BusSelector  OutputSignals=freq_bus,freq_line,wt_bus,wt_line
  Demux : Demux  Outputs=3
  Demux1 : Demux  Outputs=3
  Demux10 : Demux  Outputs=2
  Freq_Comparator : Subsystem
  Logical Operator : Logic  Inputs=3  AllPortsSameDT=off  OutDataTypeStr=boolean
  Logical Operator3 : Logic  Operator=OR  AllPortsSameDT=off  OutDataTypeStr=boolean
  Mux1 : Mux  Inputs=2
  Phase_Comparator : Subsystem
  Scope{,1..3} (4 alike) : Scope  NumInputPorts=3
  Terminator{5..8} (4 alike) : Terminator
  Voltage_Comparator : Subsystem
  deadbus fcn : MATLAB Function  TreatAsAtomicUnit=on
  dMeas : Outport
  R25 : Outport  Port=2
  wires:
  Bus Creator/1 -> dMeas/1
  Phase_Comparator/2(dWt) -> Bus Creator/1  "dWt"
  Freq_Comparator/2(dF) -> Bus Creator/2  "dF"
  Voltage_Comparator/2(dV) -> Bus Creator/3  "dV"
  [dV_threshold] -> Scope1/3, Voltage_Comparator/3(dV_threshold)
  [angle_threshold] -> Scope3/3, Phase_Comparator/3(angle_threshold)
  [dF_threshold] -> Scope2/3, Freq_Comparator/3(dF_threshold)
  Bus Selector/4 -> [dF_threshold]  "<dF_threshold>"
  Bus Selector/3 -> [angle_threshold]  "<angle_threshold>"
  Bus Selector/2 -> [dV_threshold]  "<dV_threshold>"
  Bus Selector/1 -> [VRMSLL]  "<VRMSLL>"
  relay_param/1 -> Bus Selector/1
  Mux1/1 -> Demux10/1  "RMSLL"
  Phase_Comparator/1(Locked) -> Scope/3, Logical Operator/3  "dW"
  Freq_Comparator/1(Locked) -> Scope/2, Logical Operator/2  "dF"
  Voltage_Comparator/1(Locked) -> Scope/1, Logical Operator/1  "dV"
  Demux10/2 -> deadbus fcn/2(Vline), Scope1/2, Voltage_Comparator/2(V_line)  "vline"
  Bus Selector1/4 -> Scope3/2, Phase_Comparator/2(wt_gen)  "<wt_line>"
  Bus Selector1/3 -> Scope3/1, Phase_Comparator/1(wt_grid)  "<wt_bus>"
  Bus Selector1/2 -> Scope2/2, Freq_Comparator/2(f_gen)  "<freq_line>"
  Bus Selector1/1 -> Scope2/1, Freq_Comparator/1(f_grid)  "<freq_bus>"
  Demux10/1 -> deadbus fcn/1(Vbus), Scope1/1, Voltage_Comparator/1(V_bus)  "vbus"
  Demux/1 -> Mux1/1  "a_sys"
  Demux1/1 -> Mux1/2
  Demux1/2 -> Terminator6/1
  Demux1/3 -> Terminator5/1
  Demux/2 -> Terminator7/1
  Demux/3 -> Terminator8/1
  VPKLN_bus/1 -> Demux/1
  VPKLN_line/1 -> Demux1/1
  deadbus fcn/1(y) -> Logical Operator3/1  "deadbus"
  Logical Operator/1 -> Logical Operator3/2  "dV&dF&dW"
  pll_data/1 -> Bus Selector1/1
  Logical Operator3/1 -> R25/1

== system Microgrid_transition_model_111821_ben/Grid Feeder Protective Relay/RMS_Calculator1 ==
  note: % Copyright (c) 2016 Massachusetts Institute of Technology
      | % Permission is hereby granted, free of charge, to any person obtaining a copy of this
      | % software and associated documentation files (the "Software"), to deal in the Software
      | % without restriction, including without limitation the rights to use, copy, modify,
      | % merge, publish, distribute, sublicense, and/or sell copies of the Software, and to
      | % permit persons to whom the Software is furnished to do so, subject to the following
      | % conditions:
      | %
      | %
      | % The above copyright notice and this permission notice shall be included in
      | % all copies or substantial portions of the Software.
      | %
      | % THE SOFTWARE IS PROVIDED "AS IS", WITHOUT WARRANTY OF ANY KIND, EXPRESS OR IMPLIED,
      | % INCLUDING BUT NOT LIMITED TO THE WARRANTIES OF MERCHANTABILITY, FITNESS FOR A
      | % PARTICULAR PURPOSE AND NONINFRINGEMENT. IN NO EVENT SHALL THE AUTHORS OR COPYRIGHT
      | % HOLDERS BE LIABLE FOR ANY CLAIM, DAMAGES OR OTHER LIABILITY, WHETHER IN AN ACTION
      | % OF CONTRACT, TORT OR OTHERWISE, ARISING FROM, OUT OF OR IN CONNECTION WITH THE
      | % SOFTWARE OR THE USE OR OTHER DEALINGS IN THE SOFTWARE.
      | %
      | %
      | %%
  s : Inport
  Abs : Abs
  Discrete Mean value6 : powerlib_extras/Discrete Measurements/Discrete  Mean value  Freq=60  Vinit=0  Ts=Ts
      settings: SourceProductBaseCode=PS
  Product3 : Product  RndMeth=Zero
  Signed Sqrt : Sqrt  SaturateOnIntegerOverflow=on
  RMS : Outport
  wires:
  Signed Sqrt/1 -> RMS/1
  Discrete Mean value6/1 -> Abs/1
  s/1 -> Product3/2, Product3/1
  Product3/1 -> Discrete Mean value6/1
  Abs/1 -> Signed Sqrt/1

== system Microgrid_transition_model_111821_ben/Grid Feeder Protective Relay/RMS_Calculator2 ==
  note: % Copyright (c) 2016 Massachusetts Institute of Technology
      | % Permission is hereby granted, free of charge, to any person obtaining a copy of this
      | % software and associated documentation files (the "Software"), to deal in the Software
      | % without restriction, including without limitation the rights to use, copy, modify,
      | % merge, publish, distribute, sublicense, and/or sell copies of the Software, and to
      | % permit persons to whom the Software is furnished to do so, subject to the following
      | % conditions:
      | %
      | %
      | % The above copyright notice and this permission notice shall be included in
      | % all copies or substantial portions of the Software.
      | %
      | % THE SOFTWARE IS PROVIDED "AS IS", WITHOUT WARRANTY OF ANY KIND, EXPRESS OR IMPLIED,
      | % INCLUDING BUT NOT LIMITED TO THE WARRANTIES OF MERCHANTABILITY, FITNESS FOR A
      | % PARTICULAR PURPOSE AND NONINFRINGEMENT. IN NO EVENT SHALL THE AUTHORS OR COPYRIGHT
      | % HOLDERS BE LIABLE FOR ANY CLAIM, DAMAGES OR OTHER LIABILITY, WHETHER IN AN ACTION
      | % OF CONTRACT, TORT OR OTHERWISE, ARISING FROM, OUT OF OR IN CONNECTION WITH THE
      | % SOFTWARE OR THE USE OR OTHER DEALINGS IN THE SOFTWARE.
      | %
      | %
      | %%
  s : Inport
  Abs : Abs
  Discrete Mean value6 : powerlib_extras/Discrete Measurements/Discrete  Mean value  Freq=60  Vinit=0  Ts=Ts
      settings: SourceProductBaseCode=PS
  Product3 : Product  RndMeth=Zero
  Signed Sqrt : Sqrt  SaturateOnIntegerOverflow=on
  RMS : Outport
  wires:
  Signed Sqrt/1 -> RMS/1
  Discrete Mean value6/1 -> Abs/1
  s/1 -> Product3/2, Product3/1
  Product3/1 -> Discrete Mean value6/1
  Abs/1 -> Signed Sqrt/1

== system Microgrid_transition_model_111821_ben/Grid Feeder Protective Relay1/CS Modified PLL ==
  note: SPS Discrete 3-phase PLL
  note: Pierre Giroux, Gilbert Sybille
      | Power System Laboratory, IREQ
      | Hydro-Quebec
      | (August 2007)
  Vabc(pu) : Inport  PortDimensions=3
  2nd-Order Filter : powerlib_extras/Discrete  Control Blocks/Discrete  2nd-Order Filter  FilterType=Lowpass  Fo=25  Zeta=0.707  Ts=Ts  Initialize=on  Vac_Init=[0 0 Finit]  Vdc_Init=Finit  PlotResponse=off  param1=[1 500 0.1]
      settings: SourceProductBaseCode=PS
  Controller : Subsystem  mask(Discrete PID Controller){Kp=Kp, Ki=Ki, Kd=Kd, Par_Limits=[Flim(2) Flim(1)]*2*pi, Init=2*pi*Finit, Ts=Ts}
      mask prompts: Kp "Proportional gain (Kp):"; Ki "Integral gain (Ki):"; Kd "Derivative gain (Kd):"; Par_Limits "Output limits: [ Upper   Lower ]"; Init "Output initial value:"; Ts "Sample time:"
      mask help: This block implements a discrete PID controller.
      mask init:
      | UpperLimit=Par_Limits(1);
      | LowerLimit=Par_Limits(2);
      | power_initmask();
      settings: OpenFcn=power_openblockproxy();
      mask Display: disp('PID');
  Discrete Rate Limiter : powerlib_extras/Discrete  Control Blocks/Discrete Rate Limiter  R=12  F=-12  Vinit=Finit  Ts=Ts
      settings: SourceProductBaseCode=PS
  Discrete Mean value : powerlib_extras/Discrete Measurements/Discrete  Mean value  Freq=60  Vinit=0  Ts=Ts
      settings: SourceProductBaseCode=PS
  Gain10 : Gain  Gain=1/2/pi  SaturateOnIntegerOverflow=on  OutDataTypeStr=Inherit: Same as input  ParamDataTypeStr=Inherit: Same as input
  Mux2 : Mux  Inputs=2
  Selector : Selector  InputPortWidth=3  IndexOptions=Index vector (dialog)  Indices=2  OutputSizes=1
  Trigonometric Function : Trigonometry
  Trigonometric Function2 : Trigonometry  Operator=cos
  Unit Delay : UnitDelay  InitialCondition=Finit  SampleTime=Ts  HasFrameUpgradeWarning=on
  VCO : Subsystem
  abc_to_dq0 Transformation : powerlib_extras/Measurements/abc_to_dq0 Transformation
      settings: SourceProductBaseCode=PS
  Freq : Outport
  wt : Outport  Port=2
  Sin_Cos : Outport  Port=3
  wires:
  Discrete Mean value/1 -> Controller/1(Error)
  Controller/1(Out) -> VCO/1(w), Gain10/1  "W"
  Vabc(pu)/1 -> abc_to_dq0 Transformation/1
  abc_to_dq0 Transformation/1 -> Selector/1
  VCO/1(theta) -> Trigonometric Function/1, Trigonometric Function2/1, wt/1
  Trigonometric Function/1 -> Mux2/1
  Trigonometric Function2/1 -> Mux2/2
  Mux2/1 -> abc_to_dq0 Transformation/2, Sin_Cos/1
  Gain10/1 -> Discrete Rate Limiter/1
  Discrete Rate Limiter/1 -> 2nd-Order Filter/1
  Unit Delay/1 -> Freq/1
  2nd-Order Filter/1 -> Unit Delay/1
  Selector/1 -> Discrete Mean value/1  "Vq"

== system Microgrid_transition_model_111821_ben/Grid Feeder Protective Relay1/CS Modified PLL1 ==
  note: SPS Discrete 3-phase PLL
  note: Pierre Giroux, Gilbert Sybille
      | Power System Laboratory, IREQ
      | Hydro-Quebec
      | (August 2007)
  Vabc(pu) : Inport  PortDimensions=3
  2nd-Order Filter : powerlib_extras/Discrete  Control Blocks/Discrete  2nd-Order Filter  FilterType=Lowpass  Fo=25  Zeta=0.707  Ts=Ts  Initialize=on  Vac_Init=[0 0 Finit]  Vdc_Init=Finit  PlotResponse=off  param1=[1 500 0.1]
      settings: SourceProductBaseCode=PS
  Controller : Subsystem  mask(Discrete PID Controller){Kp=Kp, Ki=Ki, Kd=Kd, Par_Limits=[Flim(2) Flim(1)]*2*pi, Init=2*pi*Finit, Ts=Ts}
      mask prompts: Kp "Proportional gain (Kp):"; Ki "Integral gain (Ki):"; Kd "Derivative gain (Kd):"; Par_Limits "Output limits: [ Upper   Lower ]"; Init "Output initial value:"; Ts "Sample time:"
      mask help: This block implements a discrete PID controller.
      mask init:
      | UpperLimit=Par_Limits(1);
      | LowerLimit=Par_Limits(2);
      | power_initmask();
      settings: OpenFcn=power_openblockproxy();
      mask Display: disp('PID');
  Discrete Rate Limiter : powerlib_extras/Discrete  Control Blocks/Discrete Rate Limiter  R=12  F=-12  Vinit=Finit  Ts=Ts
      settings: SourceProductBaseCode=PS
  Discrete Mean value : powerlib_extras/Discrete Measurements/Discrete  Mean value  Freq=60  Vinit=0  Ts=Ts
      settings: SourceProductBaseCode=PS
  Gain10 : Gain  Gain=1/2/pi  SaturateOnIntegerOverflow=on  OutDataTypeStr=Inherit: Same as input  ParamDataTypeStr=Inherit: Same as input
  Mux2 : Mux  Inputs=2
  Selector : Selector  InputPortWidth=3  IndexOptions=Index vector (dialog)  Indices=2  OutputSizes=1
  Trigonometric Function : Trigonometry
  Trigonometric Function2 : Trigonometry  Operator=cos
  Unit Delay : UnitDelay  InitialCondition=Finit  SampleTime=Ts  HasFrameUpgradeWarning=on
  VCO : Subsystem
  abc_to_dq0 Transformation : powerlib_extras/Measurements/abc_to_dq0 Transformation
      settings: SourceProductBaseCode=PS
  Freq : Outport
  wt : Outport  Port=2
  Sin_Cos : Outport  Port=3
  wires:
  Discrete Mean value/1 -> Controller/1(Error)
  Controller/1(Out) -> VCO/1(w), Gain10/1  "W"
  Vabc(pu)/1 -> abc_to_dq0 Transformation/1
  abc_to_dq0 Transformation/1 -> Selector/1
  VCO/1(theta) -> Trigonometric Function/1, Trigonometric Function2/1, wt/1
  Trigonometric Function/1 -> Mux2/1
  Trigonometric Function2/1 -> Mux2/2
  Mux2/1 -> abc_to_dq0 Transformation/2, Sin_Cos/1
  Gain10/1 -> Discrete Rate Limiter/1
  Discrete Rate Limiter/1 -> 2nd-Order Filter/1
  Unit Delay/1 -> Freq/1
  2nd-Order Filter/1 -> Unit Delay/1
  Selector/1 -> Discrete Mean value/1  "Vq"

== system Microgrid_transition_model_111821_ben/Grid Feeder Protective Relay1/R25 - Sync Check v0.1 ==
  note: Copyright 2018 Alliance for Sustainable Energy, LLC
      |
      | Permission is hereby granted, free of charge, to any person obtaining a copy of this software
      | and associated documentation files (the "Software"), to deal in the Software without restriction,
      | including without limitation the rights to use, copy, modify, merge, publish, distribute, sublicense,
      | and/or sell copies of the Software, and to permit persons to whom the Software is furnished to do so,
      | subject to the following conditions:
      |
      | The above copyright notice and this permission notice shall be included in all copies or substantial portions of the Software.
      |
      | THE SOFTWARE IS PROVIDED "AS IS", WITHOUT WARRANTY OF ANY KIND, EXPRESS OR IMPLIED, INCLUDING
      | BUT NOT LIMITED TO THE WARRANTIES OF MERCHANTABILITY, FITNESS FOR A PARTICULAR PURPOSE AND
      | NONINFRINGEMENT. IN NO EVENT SHALL THE AUTHORS, THE COPYRIGHT HOLDERS, THE UNITED STATES,
      | THE UNITED STATES DEPARTMENT OF ENERGY, OR ANY OF THEIR EMPLOYEES BE LIABLE FOR ANY CLAIM,
      | DAMAGES OR OTHER LIABILITY, WHETHER IN AN ACTION OF CONTRACT, TORT OR OTHERWISE, ARISING FROM,
      | OUT OF OR IN CONNECTION WITH THE SOFTWARE OR THE USE OR OTHER DEALINGS IN THE SOFTWARE.
  note: true: If the life bus has voltage > 0.9pu and the other bus has voltage < threshold
      | true: both sides of the breaker are deadbuses
  note: voltage difference
  note: frequency difference
  note: angle difference
  note: * this block checks for synchronism based on phase A only
      | * the block also implements a deadbus logic
  VPKLN_bus : Inport
  VPKLN_line : Inport  Port=2
  pll_data : Inport  Port=3
  relay_param : Inport  Port=4
  Bus Creator : BusCreator  Inputs=3
  Bus Selector : BusSelector  OutputSignals=VRMSLL,dV_threshold,angle_threshold,dF_threshold
  Bus Selector1 : BusSelector  OutputSignals=freq_bus,freq_line,wt_bus,wt_line
  Demux : Demux  Outputs=3
  Demux1 : Demux  Outputs=3
  Demux10 : Demux  Outputs=2
  Freq_Comparator : Subsystem
  Logical Operator : Logic  Inputs=3  AllPortsSameDT=off  OutDataTypeStr=boolean
  Logical Operator3 : Logic  Operator=OR  AllPortsSameDT=off  OutDataTypeStr=boolean
  Mux1 : Mux  Inputs=2
  Phase_Comparator : Subsystem
  Scope{,1..3} (4 alike) : Scope  NumInputPorts=3
  Terminator{5..8} (4 alike) : Terminator
  Voltage_Comparator : Subsystem
  deadbus fcn : MATLAB Function  TreatAsAtomicUnit=on
  dMeas : Outport
  R25 : Outport  Port=2
  wires:
  Logical Operator3/1 -> R25/1
  pll_data/1 -> Bus Selector1/1
  Logical Operator/1 -> Logical Operator3/2  "dV&dF&dW"
  deadbus fcn/1(y) -> Logical Operator3/1  "deadbus"
  VPKLN_line/1 -> Demux1/1
  VPKLN_bus/1 -> Demux/1
  Demux/3 -> Terminator8/1
  Demux/2 -> Terminator7/1
  Demux1/3 -> Terminator5/1
  Demux1/2 -> Terminator6/1
  Demux1/1 -> Mux1/2
  Demux/1 -> Mux1/1  "a_sys"
  Mux1/1 -> Demux10/1  "RMSLL"
  relay_param/1 -> Bus Selector/1
  Bus Selector/1 -> [VRMSLL]  "<VRMSLL>"
  Bus Selector/2 -> [dV_threshold]  "<dV_threshold>"
  Bus Selector/3 -> [angle_threshold]  "<angle_threshold>"
  Bus Selector/4 -> [dF_threshold]  "<dF_threshold>"
  Voltage_Comparator/2(dV) -> Bus Creator/3  "dV"
  Freq_Comparator/2(dF) -> Bus Creator/2  "dF"
  Phase_Comparator/2(dWt) -> Bus Creator/1  "dWt"
  Bus Creator/1 -> dMeas/1
  Freq_Comparator/1(Locked) -> Scope/2, Logical Operator/2  "dF"
  Voltage_Comparator/1(Locked) -> Scope/1, Logical Operator/1  "dV"
  Phase_Comparator/1(Locked) -> Scope/3, Logical Operator/3  "dW"
  [dV_threshold] -> Voltage_Comparator/3(dV_threshold), Scope1/3
  Demux10/1 -> Scope1/1, Voltage_Comparator/1(V_bus), deadbus fcn/1(Vbus)  "vbus"
  Demux10/2 -> Scope1/2, Voltage_Comparator/2(V_line), deadbus fcn/2(Vline)  "vline"
  Bus Selector1/1 -> Scope2/1, Freq_Comparator/1(f_grid)  "<freq_bus>"
  Bus Selector1/2 -> Scope2/2, Freq_Comparator/2(f_gen)  "<freq_line>"
  [dF_threshold] -> Scope2/3, Freq_Comparator/3(dF_threshold)
  [angle_threshold] -> Scope3/3, Phase_Comparator/3(angle_threshold)
  Bus Selector1/4 -> Scope3/2, Phase_Comparator/2(wt_gen)  "<wt_line>"
  Bus Selector1/3 -> Scope3/1, Phase_Comparator/1(wt_grid)  "<wt_bus>"

== system Microgrid_transition_model_111821_ben/Grid Feeder Protective Relay1/RMS_Calculator1 ==
  note: % Copyright (c) 2016 Massachusetts Institute of Technology
      | % Permission is hereby granted, free of charge, to any person obtaining a copy of this
      | % software and associated documentation files (the "Software"), to deal in the Software
      | % without restriction, including without limitation the rights to use, copy, modify,
      | % merge, publish, distribute, sublicense, and/or sell copies of the Software, and to
      | % permit persons to whom the Software is furnished to do so, subject to the following
      | % conditions:
      | %
      | %
      | % The above copyright notice and this permission notice shall be included in
      | % all copies or substantial portions of the Software.
      | %
      | % THE SOFTWARE IS PROVIDED "AS IS", WITHOUT WARRANTY OF ANY KIND, EXPRESS OR IMPLIED,
      | % INCLUDING BUT NOT LIMITED TO THE WARRANTIES OF MERCHANTABILITY, FITNESS FOR A
      | % PARTICULAR PURPOSE AND NONINFRINGEMENT. IN NO EVENT SHALL THE AUTHORS OR COPYRIGHT
      | % HOLDERS BE LIABLE FOR ANY CLAIM, DAMAGES OR OTHER LIABILITY, WHETHER IN AN ACTION
      | % OF CONTRACT, TORT OR OTHERWISE, ARISING FROM, OUT OF OR IN CONNECTION WITH THE
      | % SOFTWARE OR THE USE OR OTHER DEALINGS IN THE SOFTWARE.
      | %
      | %
      | %%
  s : Inport
  Abs : Abs
  Discrete Mean value6 : powerlib_extras/Discrete Measurements/Discrete  Mean value  Freq=60  Vinit=0  Ts=Ts
      settings: SourceProductBaseCode=PS
  Product3 : Product  RndMeth=Zero
  Signed Sqrt : Sqrt  SaturateOnIntegerOverflow=on
  RMS : Outport
  wires:
  Abs/1 -> Signed Sqrt/1
  Product3/1 -> Discrete Mean value6/1
  s/1 -> Product3/1, Product3/2
  Discrete Mean value6/1 -> Abs/1
  Signed Sqrt/1 -> RMS/1
